simulink model "Appl_PaComfort_CtrlModel"  (R2018b)
settings: configuration reference "CodeConfig_10_ms" (kept outside this file)
undefined symbols (not defined in the file): D_CLOSE, D_InitDelayTime, D_OPEN, D_SoftDistancePaLegnth, D_WelcomeDistance, FALSE, TRUE
libraries: DareLib x44, simulink x1
(part 2 of 2)

== stateflow chart Appl_PaComfort_CtrlModel/UpDataInputInfo/InputSignalProcess/WelcomePRM/ComfortDeal ==
  state SetComfortPrm(in) [function]
  state Init
    en:
    InitTimer = 1;
    ComfortOpenFlag = FALSE;
    ComfortOpenMsg = TRUE;
    du:
    InitTimer ++;
    ex:
    InitTimer = 0;
  state Configurable
    state Enable
      en:
      ComfortOpenFlag = TRUE;
      /**ComfortOpenMsg 报文发送变量****************ComfortOpenFlag迎宾功能是否开启变量即PC1迎宾功能处于开启状态*/
      SetComfortPrm(TRUE);
      ComfortOpenMsg = TRUE;
    state Disable
      en:
      ComfortOpenFlag = FALSE;
      SetComfortPrm(FALSE);
      ComfortOpenMsg = FALSE;
    (junction 73) -> Enable [order 1] : [MtrWel_WelcomeSwitch == 1]
    Enable -> Disable : /*当IVI_St_FLSeatmeet=0x2:Close时，座椅调节舒适进入禁能*/
        | [2 == MtrWel_0x351_IVI_St_FLSeatmeet]
    Disable -> Enable : /*当IVI_St_FLSeatmeet=0x1:Open时，座椅调节舒适进入使能*/
        | [1 == MtrWel_0x351_IVI_St_FLSeatmeet]
    (default) -> (junction 73)
    (junction 73) -> Disable [order 2]
  (default) -> Init
  Init -> Configurable : /*EEPROM迎宾为使能&&座椅电动调节&&P20车型&&初始化完成&&正常电压*/
      | [TRUE == MtrWel_WelcomeEnable ...
      | && (enDrAdjustEnable.EN_DrSixWayMotor == MtrWel_AdjustEnable ...
      | || enDrAdjustEnable.EN_DrTwelveWayMotor == MtrWel_AdjustEnable) ...
      | && enVehTypePrm.enP20 == MtrWel_VehiclePrm ...
      | && InitTimer > D_InitDelayTime ...
      | && enFinalPowerMode.EN_NORMAL_VOLT == MtrWel_VoltMode]
  Configurable -> Init [order 1] : /*恢复出厂设置*/
      | [TRUE == MtrWel_GetRecoverDefaultFlag]
      | /SetComfortPrm(TRUE);
  Configurable -> Init [order 2] : /*((迎宾禁能 || 座椅为手动调节 || 电压非正常模式)&&P20车型)
      | || 非P20车型*/
      | [((TRUE != MtrWel_WelcomeEnable ...
      | || enDrAdjustEnable.EN_DrManual  == MtrWel_AdjustEnable ...
      | || enFinalPowerMode.EN_NORMAL_VOLT != MtrWel_VoltMode) ...
      | && enVehTypePrm.enP20 == MtrWel_VehiclePrm) ...
      | || enVehTypePrm.enP20 != MtrWel_VehiclePrm]
  data: in function_input; MtrWel_0x351_IVI_St_FLSeatmeet input; MtrWel_WelcomeEnable input; ComfortOpenFlag output uint8; TRUE parameter; FALSE parameter; InitTimer local uint8; MtrWel_VoltMode input; MtrWel_AdjustEnable input; MtrWel_VehiclePrm input; MtrWel_WelcomeSwitch input; D_InitDelayTime parameter; MtrWel_GetRecoverDefaultFlag input; ComfortOpenMsg output uint8
